simulink model "test_state_space"  (Simulink 7.6)
settings: Solver=ode45  StartTime=0.0  StopTime=0.2  MaxStep=0.01  RelTol=1e-3
settings Model: Creator=guillaume.laurent  LastModifiedBy=guillaume.laurent
settings DebuggingCC: StrictBusMsg=Warning

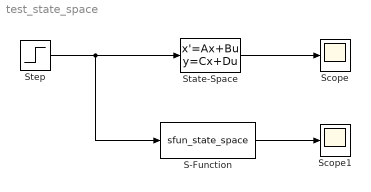
== system test_state_space ==
  S-Function : S-Function  FunctionName=sfun_state_space  Parameters="[ -0.09  -0.01 ;  1   ,  0   ]  [  1    -7  ;   0   , -2   ] [  0    2  ;  1   , -5   ] [ -3   0   ;   1   , 0     ]"  EnableBusSupport=off
  Scope : Scope
  Scope1 : Scope
  State-Space : StateSpace  A="[ -0.09  -0.01 ;  1   ,  0   ]"  B="[  1    -7  ;   0   , -2   ]"  C="[  0    2  ;  1   , -5   ]"  D="[ -3   0   ;   1   , 0     ]"
  Step : Step  Time=0.1  Before=[0 0]  After=[1 1]  SampleTime=0
  wires:
  Step/1 -> State-Space/1, S-Function/1
  State-Space/1 -> Scope/1
  S-Function/1 -> Scope1/1
